simulink model "ARI_24_8_DOF2"  (Simulink 7.8)
settings: Solver=ode45  SolverMode=SingleTasking  StartTime=0.0  StopTime=10  RelTol=1e-10  AbsTol=1e-10
values from neighbouring files (symbols this model uses):
  h = findobj(gcf,'type','line')    [boldLines.m]    (also in phase.m = min(hmax, 0.9*h*(tau/delta)^pow))
  p = plot(x,y,'b.',0,0,'g*','EraseMode','none','MarkerSize',10);hold on    [PAplot.m]
undefined symbols (not defined in the file or in its folder): A, B, C, D
libraries: simulink x1
settings Model: Creator=Michael Sebek  ModifiedByFormat=Michael Sebek  LastModifiedBy=Michael Sebek  ExtModeTrigMode=oneshot  ExtModeArmWhenConnect=off
settings DataIOCC: LimitDataPoints=off
settings OptimizationCC: BlockReduction=off  BooleanDataType=off  InitFltsAndDblsToZero=on
settings DebuggingCC: SaveWithParameterizedLinksMsg=none  SignalResolutionControl=TryResolveAllWithWarning  SolverPrmCheckMsg=none  MultiTaskDSMMsg=warning  MultiTaskCondExecSysMsg=none  FcnCallInpInsideContextMsg=Use local settings  StrictBusMsg=None
settings HardwareCC: TargetUnknown=on
settings RTWCC: IncludeERTFirstTime=on
settings GRTTargetCC: TargetFcnLib=ansi_tfl_tmw.mat

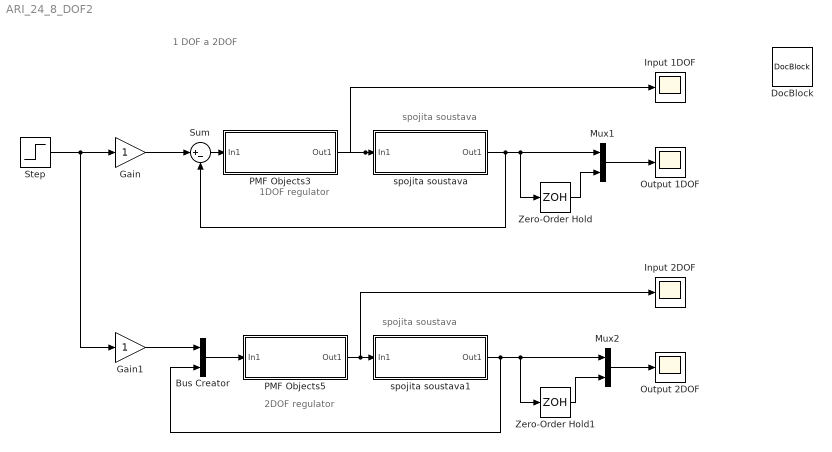
== system ARI_24_8_DOF2 ==
  note: 1 DOF a 2DOF
  note: spojita soustava
  note: 1DOF regulator
  note: spojita soustava
  note: 2DOF regulator
  Bus Creator : BusCreator  Inputs=2
  DocBlock : simulink/Model-Wide Utilities/DocBlock  DocumentType=Text
  Gain : Gain
  Gain1 : Gain
  Input 1DOF : Scope
      settings: TickLabels=on  TimeRange=2  YMin=-2000  YMax=2000  DataFormat=Array
  Input 2DOF : Scope
      settings: TickLabels=on  TimeRange=2  YMin=-2000  YMax=2000  DataFormat=Array
  Mux1 : Mux  Inputs=2
  Mux2 : Mux  Inputs=2
  Output 1DOF : Scope
      settings: TickLabels=on  TimeRange=2  YMin=-3  YMax=3  DataFormat=Array
  Output 2DOF : Scope
      settings: TickLabels=on  TimeRange=2  YMin=-1  YMax=3  SaveName=ScopeData2  DataFormat=Array
  PMF Objects3 : Subsystem  mask(PMF Block){F=q/p, InCon=[ ], SampTime=h, fvar=No change}
      mask prompts: F "PMF Object:"; InCon "Initial states:"; SampTime "Sample time (discrete time only):"; fvar "Force variable:"
      mask help:
      | Polynomial matrix fraction description of a linear system.
      |
      | This block represents a linear system defined by the polynomial matrix fraction of its transfer function.
      mask init:
      | Label = 'xxx';
      | [A,B,C,D,Label,var] = polymask2(F, fvar, length(InCon));
      | update;
      mask Help:
      | This block represents a linear system [<I>A,B,C,D</I>] defined by the polynomial matrix fraction (<I>PMF</I>) of its transfer function <I>T</I>.
      | <p>
      | <b>Left Matrix Fraction</b> item of the popup menu <b>Type</b> indicates the transfer function in the form of <I>left PMF</I>:
      | <p>
      | <I>T</I> = inv(<I>Q</I>) <I>P</I>.
      | <p>
      | <b>Right Matrix Fraction</b> item is used if the transfer function is given in the form of <I>right PMF</I>:
      | <p>
      | <I>T</I> = <I>P</I> inv(<I>Q</I>).
      | <p>
      |  The <b>variable</b> determines the type  of the system:
      | <p>
      | - <b>s, p</b> are used for continous time systems (Laplace transform).
      | <p>
      | - <b>z, q</b> are used for discrete time transfer functions in forward-shift operator (Z-transform).
      | <p>
      | - <b>d, z^-1</b> are used for discrete time transfer functions in backward-shift operator.
      | <p>
      | <b> Note:</b> For the variables <I>s,p,z,q</I>, the transfer function is defined as
      | <p>
      | <I>T</I> = <I>C</I> inv(<I>vI-A</I>) <I>B</I> + <I>D</I>,
      | <p>
      | where <I>v</I> is the variable of <I>P,Q</I>.
      | For the variables <I>d, z^-1</I>, the transfer function is defined as
      | <p>
      | <I>T</I> = <I>C v</I> inv(<I>I-Av</I>)  <I>B</I> + <I>D</I>.
      | <p>
      | <b>Note:</b> <b>Initial states</b> concern the observer-form realization of the system as defined by LMF2S and RMF2S functions. Their number must equal the sum of column degrees of the denominator matrix <I>Q</I> in case of right PMF and the sum of row degrees of <I>Q</I> for left PMF description.
      | <p>
      | See also POL, LMF2S, RMF2S.
      mask StyleString: edit,edit,edit,popup(No change|s   (continous time)|p   (continous time)|z      (discrete time)|q      (discrete time)|d      (discrete time)|z^-1 (discrete time))
      mask Display: disp(Label);
  PMF Objects5 : Subsystem  mask(PMF Block){F=[r -q]/p, InCon=[ ], SampTime=h, fvar=No change}
      mask prompts: F "PMF Object:"; InCon "Initial states:"; SampTime "Sample time (discrete time only):"; fvar "Force variable:"
      mask help:
      | Polynomial matrix fraction description of a linear system.
      |
      | This block represents a linear system defined by the polynomial matrix fraction of its transfer function.
      mask init:
      | Label = 'xxx';
      | [A,B,C,D,Label,var] = polymask2(F, fvar, length(InCon));
      | update;
      mask Help:
      | This block represents a linear system [<I>A,B,C,D</I>] defined by the polynomial matrix fraction (<I>PMF</I>) of its transfer function <I>T</I>.
      | <p>
      | <b>Left Matrix Fraction</b> item of the popup menu <b>Type</b> indicates the transfer function in the form of <I>left PMF</I>:
      | <p>
      | <I>T</I> = inv(<I>Q</I>) <I>P</I>.
      | <p>
      | <b>Right Matrix Fraction</b> item is used if the transfer function is given in the form of <I>right PMF</I>:
      | <p>
      | <I>T</I> = <I>P</I> inv(<I>Q</I>).
      | <p>
      |  The <b>variable</b> determines the type  of the system:
      | <p>
      | - <b>s, p</b> are used for continous time systems (Laplace transform).
      | <p>
      | - <b>z, q</b> are used for discrete time transfer functions in forward-shift operator (Z-transform).
      | <p>
      | - <b>d, z^-1</b> are used for discrete time transfer functions in backward-shift operator.
      | <p>
      | <b> Note:</b> For the variables <I>s,p,z,q</I>, the transfer function is defined as
      | <p>
      | <I>T</I> = <I>C</I> inv(<I>vI-A</I>) <I>B</I> + <I>D</I>,
      | <p>
      | where <I>v</I> is the variable of <I>P,Q</I>.
      | For the variables <I>d, z^-1</I>, the transfer function is defined as
      | <p>
      | <I>T</I> = <I>C v</I> inv(<I>I-Av</I>)  <I>B</I> + <I>D</I>.
      | <p>
      | <b>Note:</b> <b>Initial states</b> concern the observer-form realization of the system as defined by LMF2S and RMF2S functions. Their number must equal the sum of column degrees of the denominator matrix <I>Q</I> in case of right PMF and the sum of row degrees of <I>Q</I> for left PMF description.
      | <p>
      | See also POL, LMF2S, RMF2S.
      mask StyleString: edit,edit,edit,popup(No change|s   (continous time)|p   (continous time)|z      (discrete time)|q      (discrete time)|d      (discrete time)|z^-1 (discrete time))
      mask Display: disp(Label);
  Step : Step  SampleTime=0
  Sum : Sum  Inputs=|+-
  Zero-Order Hold : ZeroOrderHold  SampleTime=h
  Zero-Order Hold1 : ZeroOrderHold  SampleTime=h
  spojita soustava : Subsystem  mask(PMF Block){F=1/s^2, InCon=[1 -1 ], SampTime=1, fvar=No change}
      mask prompts: F "PMF Object:"; InCon "Initial states:"; SampTime "Sample time (discrete time only):"; fvar "Force variable:"
      mask help:
      | Polynomial matrix fraction description of a linear system.
      |
      | This block represents a linear system defined by the polynomial matrix fraction of its transfer function.
      mask init:
      | Label = 'xxx';
      | [A,B,C,D,Label,var] = polymask2(F, fvar, length(InCon));
      | update;
      mask Help:
      | This block represents a linear system [<I>A,B,C,D</I>] defined by the polynomial matrix fraction (<I>PMF</I>) of its transfer function <I>T</I>.
      | <p>
      | <b>Left Matrix Fraction</b> item of the popup menu <b>Type</b> indicates the transfer function in the form of <I>left PMF</I>:
      | <p>
      | <I>T</I> = inv(<I>Q</I>) <I>P</I>.
      | <p>
      | <b>Right Matrix Fraction</b> item is used if the transfer function is given in the form of <I>right PMF</I>:
      | <p>
      | <I>T</I> = <I>P</I> inv(<I>Q</I>).
      | <p>
      |  The <b>variable</b> determines the type  of the system:
      | <p>
      | - <b>s, p</b> are used for continous time systems (Laplace transform).
      | <p>
      | - <b>z, q</b> are used for discrete time transfer functions in forward-shift operator (Z-transform).
      | <p>
      | - <b>d, z^-1</b> are used for discrete time transfer functions in backward-shift operator.
      | <p>
      | <b> Note:</b> For the variables <I>s,p,z,q</I>, the transfer function is defined as
      | <p>
      | <I>T</I> = <I>C</I> inv(<I>vI-A</I>) <I>B</I> + <I>D</I>,
      | <p>
      | where <I>v</I> is the variable of <I>P,Q</I>.
      | For the variables <I>d, z^-1</I>, the transfer function is defined as
      | <p>
      | <I>T</I> = <I>C v</I> inv(<I>I-Av</I>)  <I>B</I> + <I>D</I>.
      | <p>
      | <b>Note:</b> <b>Initial states</b> concern the observer-form realization of the system as defined by LMF2S and RMF2S functions. Their number must equal the sum of column degrees of the denominator matrix <I>Q</I> in case of right PMF and the sum of row degrees of <I>Q</I> for left PMF description.
      | <p>
      | See also POL, LMF2S, RMF2S.
      mask StyleString: edit,edit,edit,popup(No change|s   (continous time)|p   (continous time)|z      (discrete time)|q      (discrete time)|d      (discrete time)|z^-1 (discrete time))
      mask Display: disp(Label);
  spojita soustava1 : Subsystem  mask(PMF Block){F=1/s^2, InCon=[1 -1 ], SampTime=1, fvar=No change}
      mask prompts: F "PMF Object:"; InCon "Initial states:"; SampTime "Sample time (discrete time only):"; fvar "Force variable:"
      mask help:
      | Polynomial matrix fraction description of a linear system.
      |
      | This block represents a linear system defined by the polynomial matrix fraction of its transfer function.
      mask init:
      | Label = 'xxx';
      | [A,B,C,D,Label,var] = polymask2(F, fvar, length(InCon));
      | update;
      mask Help:
      | This block represents a linear system [<I>A,B,C,D</I>] defined by the polynomial matrix fraction (<I>PMF</I>) of its transfer function <I>T</I>.
      | <p>
      | <b>Left Matrix Fraction</b> item of the popup menu <b>Type</b> indicates the transfer function in the form of <I>left PMF</I>:
      | <p>
      | <I>T</I> = inv(<I>Q</I>) <I>P</I>.
      | <p>
      | <b>Right Matrix Fraction</b> item is used if the transfer function is given in the form of <I>right PMF</I>:
      | <p>
      | <I>T</I> = <I>P</I> inv(<I>Q</I>).
      | <p>
      |  The <b>variable</b> determines the type  of the system:
      | <p>
      | - <b>s, p</b> are used for continous time systems (Laplace transform).
      | <p>
      | - <b>z, q</b> are used for discrete time transfer functions in forward-shift operator (Z-transform).
      | <p>
      | - <b>d, z^-1</b> are used for discrete time transfer functions in backward-shift operator.
      | <p>
      | <b> Note:</b> For the variables <I>s,p,z,q</I>, the transfer function is defined as
      | <p>
      | <I>T</I> = <I>C</I> inv(<I>vI-A</I>) <I>B</I> + <I>D</I>,
      | <p>
      | where <I>v</I> is the variable of <I>P,Q</I>.
      | For the variables <I>d, z^-1</I>, the transfer function is defined as
      | <p>
      | <I>T</I> = <I>C v</I> inv(<I>I-Av</I>)  <I>B</I> + <I>D</I>.
      | <p>
      | <b>Note:</b> <b>Initial states</b> concern the observer-form realization of the system as defined by LMF2S and RMF2S functions. Their number must equal the sum of column degrees of the denominator matrix <I>Q</I> in case of right PMF and the sum of row degrees of <I>Q</I> for left PMF description.
      | <p>
      | See also POL, LMF2S, RMF2S.
      mask StyleString: edit,edit,edit,popup(No change|s   (continous time)|p   (continous time)|z      (discrete time)|q      (discrete time)|d      (discrete time)|z^-1 (discrete time))
      mask Display: disp(Label);
  wires:
  spojita soustava/1(Out1) -> Zero-Order Hold/1, Mux1/1, Sum/2
  Mux1/1 -> Output 1DOF/1
  Zero-Order Hold/1 -> Mux1/2
  Sum/1 -> PMF Objects3/1(In1)
  PMF Objects3/1(Out1) -> spojita soustava/1(In1), Input 1DOF/1
  Gain/1 -> Sum/1
  Step/1 -> Gain/1, Gain1/1
  spojita soustava1/1(Out1) -> Mux2/1, Zero-Order Hold1/1, Bus Creator/2
  Mux2/1 -> Output 2DOF/1
  Zero-Order Hold1/1 -> Mux2/2
  Gain1/1 -> Bus Creator/1
  Bus Creator/1 -> PMF Objects5/1(In1)
  PMF Objects5/1(Out1) -> spojita soustava1/1(In1), Input 2DOF/1

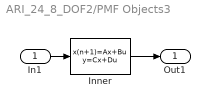
== system ARI_24_8_DOF2/PMF Objects3 ==
  In1 : Inport
  Inner : DiscreteStateSpace  A=A  B=B  C=C  D=D  X0=InCon  SampleTime=SampTime
  Out1 : Outport
  wires:
  In1/1 -> Inner/1
  Inner/1 -> Out1/1

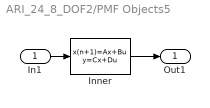
== system ARI_24_8_DOF2/PMF Objects5 ==
  In1 : Inport
  Inner : DiscreteStateSpace  A=A  B=B  C=C  D=D  X0=InCon  SampleTime=SampTime
  Out1 : Outport
  wires:
  Inner/1 -> Out1/1
  In1/1 -> Inner/1

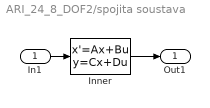
== system ARI_24_8_DOF2/spojita soustava ==
  In1 : Inport
  Inner : StateSpace  A=A  B=B  C=C  D=D  X0=InCon
  Out1 : Outport
  wires:
  Inner/1 -> Out1/1
  In1/1 -> Inner/1

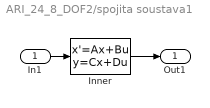
== system ARI_24_8_DOF2/spojita soustava1 ==
  In1 : Inport
  Inner : StateSpace  A=A  B=B  C=C  D=D  X0=InCon
  Out1 : Outport
  wires:
  In1/1 -> Inner/1
  Inner/1 -> Out1/1
